simulink model "PFV_rooftop"  (R2017a)
settings: Solver=ode23s  StartTime=0.0  StopTime=0.5  MaxStep=1e-6
libraries: powerlib x16, simulink x4
settings Model: Creator=sibly  LastModifiedBy=alfonso

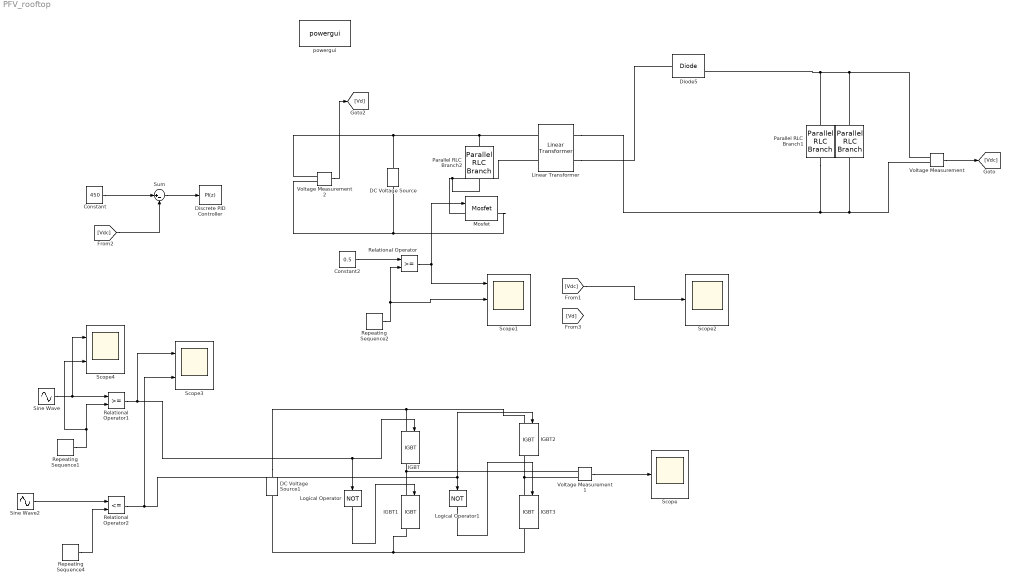
== system PFV_rooftop ==
  " " : powerlib/Elements/Parallel RLC Branch  LConnTagsString=a  RConnTagsString=__new0  BranchType=R  Resistance=450*450/500  Inductance=1e-3  SetiL0=off  InitialCurrent=0  Capacitance=1e-6  Setx0=off  InitialVoltage=0  Measurements=None
  Constant : Constant  Value=450
  Constant2 : Constant  Value=0.5
  DC Voltage Source : powerlib/Electrical Sources/DC Voltage Source  Amplitude=60  Measurements=None
  DC Voltage Source1 : powerlib/Electrical Sources/DC Voltage Source  Amplitude=450  Measurements=None
  Diode5 : powerlib/Power Electronics/Diode  Ron=0.001  Lon=0  Vf=0.8  IC=0  UseSnubber=0  Rs=500  Cs=250e-9  Measurements=on
  Discrete PID Controller : simulink/Continuous/PID Controller  Controller=PI  TimeDomain=Discrete-time  SampleTime=1/40000  IntegratorMethod=Forward Euler  FilterMethod=Forward Euler  Form=Parallel  UseFilter=on  ControllerParametersSource=internal  P=5e-04  I=0.01  D=0  N=100  InitialConditionSource=internal  InitialConditionForIntegrator=0  InitialConditionForFilter=0  ExternalReset=none  LimitOutput=off  UpperSaturationLimit=inf  LowerSaturationLimit=-inf  LinearizeAsGain=off  AntiWindupMode=none  Kb=1  TrackingMode=off  Kt=1  PParamMin=[]  PParamMax=[]  IParamMin=[]  IParamMax=[]  DParamMin=[]  DParamMax=[]  NParamMin=[]  NParamMax=[]  KbParamMin=[]  KbParamMax=[]  KtParamMin=[]  KtParamMax=[]  POutMin=[]  POutMax=[]  IOutMin=[]  IOutMax=[]  DOutMin=[]  DOutMax=[]  NOutMin=[]  NOutMax=[]  KbOutMin=[]  KbOutMax=[]  KtOutMin=[]  KtOutMax=[]  IntegratorOutMin=[]  IntegratorOutMax=[]  FilterOutMin=[]  FilterOutMax=[]  SumOutMin=[]  SumOutMax=[]  SumI1OutMin=[]  SumI1OutMax=[]  SumI2OutMin=[]  SumI2OutMax=[]  SumI3OutMin=[]  SumI3OutMax=[]  SumDOutMin=[]  SumDOutMax=[]  SaturationOutMin=[]  SaturationOutMax=[]  IntegratorContinuousStateAttributes=''  IntegratorStateMustResolveToSignalObject=off  IntegratorRTWStateStorageClass=Auto  FilterContinuousStateAttributes=''  FilterStateMustResolveToSignalObject=off  FilterRTWStateStorageClass=Auto  DifferentiatorICPrevScaledInput=0  DifferentiatorOutMin=[]  DifferentiatorOutMax=[]  InitialConditionSetting=State (most efficient)
  IGBT{,1..3} (4 alike) : powerlib/Power Electronics/IGBT  Ron=0.001  Lon=0  Vf=1  Tf=1e-6  Tt=2e-6  IC=0  Rs=1e5  Cs=inf  Measurements=on
  Linear Transformer : powerlib/Elements/Linear Transformer  UNITS=SI  NominalPower=[ 500 50 ]  winding1=[60 0 0]  winding2=[475 0 0]  ThreeWindings=off  winding3=[3.15e+05 315.06 0.12769]  RmLm=[2.3346e+09 0]  Measurements=Winding currents  DataType=on
  Logical Operator : Logic  Operator=NOT  AllPortsSameDT=off  OutDataTypeStr=boolean
  Logical Operator1 : Logic  Operator=NOT  AllPortsSameDT=off  OutDataTypeStr=boolean
  Mosfet : powerlib/Power Electronics/Mosfet  Ron=0.1  Lon=0  Rd=0.01  Vfd=0  IC=0  Rs=1e5  Cs=inf  Measurements=on
  Parallel RLC Branch1 : powerlib/Elements/Parallel RLC Branch  LConnTagsString=a  RConnTagsString=__new0  BranchType=C  Resistance=1  Inductance=1e-3  SetiL0=off  InitialCurrent=0  Capacitance=1e-3  Setx0=off  InitialVoltage=0  Measurements=None
  Parallel RLC Branch2 : powerlib/Elements/Parallel RLC Branch  LConnTagsString=a  RConnTagsString=__new0  BranchType=L  Resistance=1  Inductance=5e-4  SetiL0=off  InitialCurrent=0  Capacitance=1.5e-2  Setx0=off  InitialVoltage=0  Measurements=None
  Relational Operator : RelationalOperator  OutDataTypeStr=boolean  RndMeth=Simplest
  Relational Operator1 : RelationalOperator  OutDataTypeStr=boolean  RndMeth=Simplest
  Relational Operator2 : RelationalOperator  Operator=<=  OutDataTypeStr=boolean  RndMeth=Simplest
  Repeating Sequence1 : simulink/Sources/Repeating Sequence  rep_seq_t=[0 50e-06 100e-06]  rep_seq_y=[-1 1 -1]
  Repeating Sequence2 : simulink/Sources/Repeating Sequence  rep_seq_t=[0 1/10000]  rep_seq_y=[0 1]
  Repeating Sequence4 : simulink/Sources/Repeating Sequence  rep_seq_t=[0 50e-06 100e-06]  rep_seq_y=[1 -1 1]
  Scope : Scope
  Scope1 : Scope  NumInputPorts=3
  Scope2 : Scope
  Scope3 : Scope  NumInputPorts=2
  Scope4 : Scope  NumInputPorts=2
  Sine Wave : Sin  Amplitude=250/450  Frequency=50*2*pi  SampleTime=0
  Sine Wave2 : Sin  Amplitude=250/450  Frequency=50*2*pi  SampleTime=0
  Sum : Sum  Inputs=|+-
  Voltage Measurement : powerlib/Measurements/Voltage Measurement  PhasorSimulation=off  OutputType=Complex  PSBequivalent=0
  Voltage Measurement1 : powerlib/Measurements/Voltage Measurement  PhasorSimulation=off  OutputType=Complex  PSBequivalent=0
  Voltage Measurement2 : powerlib/Measurements/Voltage Measurement  PhasorSimulation=off  OutputType=Complex  PSBequivalent=0
  powergui : powerlib/powergui  Priority=1  SimulationMode=Continuous  SampleTime=50e-6  frequency=60  Iterations=50  frequencyindice=0  Pbase=100e6  ErrMax=1e-4  UnitsV=kV  UnitsW=MW  buscounter=0  FunctionMessages=off  echomessages=off  EnableUseOfTLC=off  CurrentSourceSwitches=off  DisableSnubberDevices=off  DisableRonSwitches=off  DisableVfSwitches=off  DisplayEquations=off  SolverType=Tustin/Backward Euler (TBE)  Interpol=off  ExternalGateDelay=off  methode=off  Ts=100  x0status=blocks  SPID=on  SwTol=0  HookPort=off  RestoreLinks=warning  ResistiveCurrentMeasurement=off  Frange=[0:2:500]  Ylog=off  Xlog=on  ShowGrid=off  save=off  variable=ZData  structure=0  ZoomFFT=off  StartTime=0.0  cycles=1  DisplayStyle=1  fundamental=60  FreqAxis=off  MaxFrequency=1000  frequencyindicesteady=1  RmsSteady=1  display=off
  wires:
  Voltage Measurement/1 -> [Vdc]
  Repeating Sequence2/1 -> Scope1/2, Relational Operator/2
  Constant/1 -> Sum/1
  [Vdc] -> Sum/2
  Sum/1 -> Discrete PID Controller/1
  Relational Operator/1 -> Scope1/1, Mosfet/1
  Voltage Measurement2/1 -> [Vd]
  [Vdc] -> Scope2/1
  Constant2/1 -> Relational Operator/1
  Relational Operator1/1 -> Scope3/1, IGBT/1, Logical Operator/1
  Repeating Sequence4/1 -> Relational Operator2/2
  Sine Wave/1 -> Scope4/1, Relational Operator1/1
  Sine Wave2/1 -> Relational Operator2/1
  Logical Operator/1 -> IGBT1/1
  Logical Operator1/1 -> IGBT3/1
  Voltage Measurement1/1 -> Scope/1
  Relational Operator2/1 -> Scope3/2, IGBT2/1, Logical Operator1/1
  Repeating Sequence1/1 -> Scope4/2, Relational Operator1/2
  connections:
  Voltage Measurement/LConn1 -- Diode5/RConn1 -- Parallel RLC Branch1/LConn1 -- " "/LConn1
  Linear Transformer/LConn1 -- Voltage Measurement2/LConn1 -- DC Voltage Source/RConn1 -- Parallel RLC Branch2/RConn1
  Linear Transformer/LConn2 -- Mosfet/LConn1 -- Parallel RLC Branch2/LConn1
  Mosfet/RConn1 -- DC Voltage Source/LConn1 -- Voltage Measurement2/LConn2
  Linear Transformer/RConn2 -- Diode5/LConn1
  Voltage Measurement/LConn2 -- Linear Transformer/RConn1 -- Parallel RLC Branch1/RConn1 -- " "/RConn1
  DC Voltage Source1/RConn1 -- IGBT2/LConn1 -- IGBT/LConn1
  Voltage Measurement1/LConn2 -- IGBT3/LConn1 -- IGBT2/RConn1
  DC Voltage Source1/LConn1 -- IGBT1/RConn1 -- IGBT3/RConn1
  Voltage Measurement1/LConn1 -- IGBT1/LConn1 -- IGBT/RConn1
